simulink model "chapter4_4_2_0424"  (Simulink 8.2)
settings: Solver=VariableStepDiscrete  StartTime=0.0  StopTime=30  FixedStep=0.01  RelTol=1e-3
libraries: Solver_SF x1, simulink x1
settings Model: Creator=xuwei  LastModifiedBy=liuho
settings ConfigurationSet: Description=SimMechanics 2G

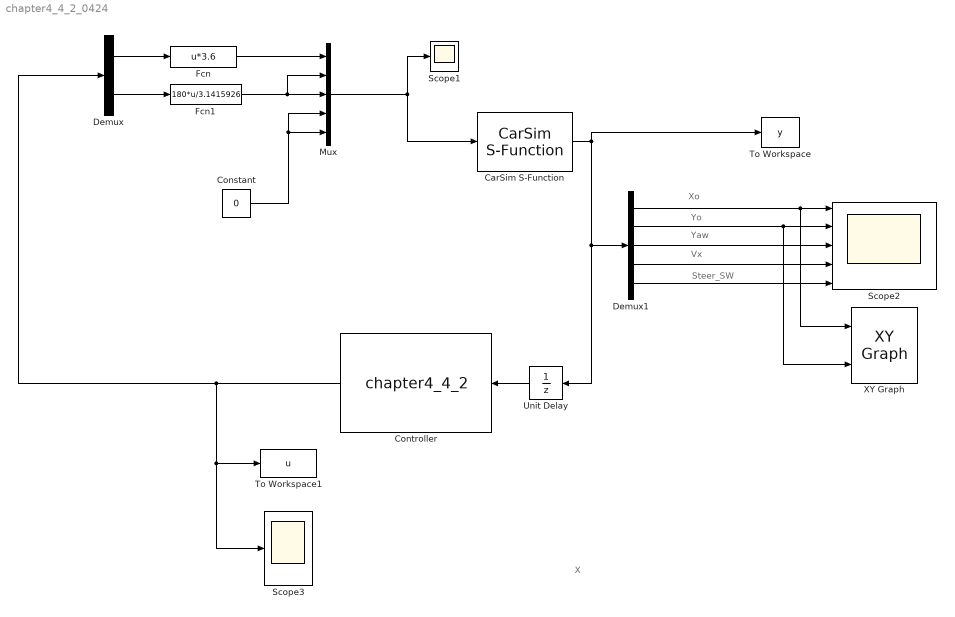
== system chapter4_4_2_0424 ==
  note: Yo
  note: Xo
  note: Yaw
  note: Vx
  note: Steer_SW
  note: X
  CarSim S-Function : Solver_SF/CarSim S-Function  Priority=1  VehicleCode=i_i  SIMFILE=LEO_MPC_EM_PathTrackingCtrl.sim
  Constant : Constant  Value=0
  Controller : S-Function  FunctionName=chapter4_4_2  EnableBusSupport=off
  Demux : Demux  Outputs=2
  Demux1 : Demux  Outputs=5
  Fcn : Fcn  Expr=u*3.6
  Fcn1 : Fcn  Expr=180*u/3.1415926
  Mux : Mux  Inputs=5
  Scope1 : Scope
      settings: SaveName=ScopeData2
  Scope2 : Scope  NumInputPorts=5
      settings: TimeRange=20  YMin=-1~35~-10~-20~-4  YMax=1~36.5~5~20~2
  Scope3 : Scope
      settings: SaveName=ScopeData3
  To Workspace : ToWorkspace  VariableName=y  SampleTime=-1  SaveFormat=Structure
  To Workspace1 : ToWorkspace  VariableName=u  SampleTime=-1  SaveFormat=Structure
  Unit Delay : UnitDelay  SampleTime=-1
  XY Graph : simulink/Sinks/XY Graph  xmin=0  xmax=500  ymin=0  ymax=20  st=-1
  wires:
  Unit Delay/1 -> Controller/1
  Mux/1 -> CarSim S-Function/1, Scope1/1
  Constant/1 -> Mux/5, Mux/4
  Fcn/1 -> Mux/1
  Fcn1/1 -> Mux/2, Mux/3
  Demux/1 -> Fcn/1
  Demux/2 -> Fcn1/1
  Controller/1 -> Demux/1, Scope3/1, To Workspace1/1
  Demux1/1 -> XY Graph/1, Scope2/1
  Demux1/2 -> XY Graph/2, Scope2/2
  Demux1/3 -> Scope2/3
  Demux1/4 -> Scope2/4
  Demux1/5 -> Scope2/5
  CarSim S-Function/1 -> Unit Delay/1, Demux1/1, To Workspace/1
